simulink model "equation_1"  (R2018b)
settings: Solver=VariableStepAuto  StartTime=0.0  StopTime=4  RelTol=1e-3
libraries: simulink x2
settings Model: Creator=dinet  LastModifiedBy=dinet

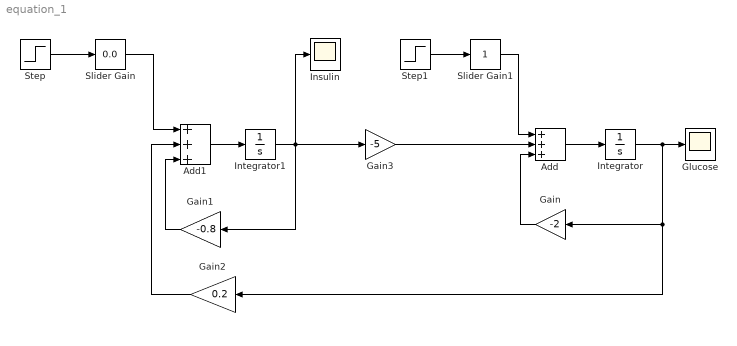
== system equation_1 ==
  Add : Sum  Inputs=+++
  Add1 : Sum  Inputs=+++
  Gain : Gain  Gain=-2
  Gain1 : Gain  Gain=-0.8
  Gain2 : Gain  Gain=0.2
  Gain3 : Gain  Gain=-5
  Glucose : Scope
  Insulin : Scope
  Integrator : Integrator
  Integrator1 : Integrator
  Slider Gain : simulink/Math Operations/Slider Gain  gain=0.0  low=0  high=2
  Slider Gain1 : simulink/Math Operations/Slider Gain  gain=1  low=0  high=2
  Step : Step  Time=0  SampleTime=0
  Step1 : Step  Time=0  SampleTime=0
  wires:
  Step/1 -> Slider Gain/1
  Slider Gain/1 -> Add1/1
  Add1/1 -> Integrator1/1
  Integrator1/1 -> Gain3/1, Insulin/1, Gain1/1
  Gain3/1 -> Add/2
  Step1/1 -> Slider Gain1/1
  Slider Gain1/1 -> Add/1
  Gain/1 -> Add/3
  Add/1 -> Integrator/1
  Integrator/1 -> Gain2/1, Gain/1, Glucose/1
  Gain1/1 -> Add1/3
  Gain2/1 -> Add1/2
